simulink model "mbd_example_qdec"  (R2022b)
settings: Solver=FixedStepDiscrete  StartTime=0.0  StopTime=10.0  RelTol=1e-3  EnableMultiTasking=on
PostLoadFcn:
  | run([bdroot '_init']);
InitFcn:
  | checkModelFolder(true); % Optional
  | run([bdroot '_init']);
model workspace (MAT data in the model file):
  MBDPortal_MaskInitParam = 0
  MBDPortal_MaskInitSignal = 0
  MBDSnap_MaskInitSignal = 0
undefined symbols (not defined in the file): MBDDiag_Comm_Module, MBDDiag_Comm_Speed, MBDDiag_Comm_Type, T_s_LED1, T_s_LED2
libraries: MbdLib_PortalDiag x24, MbdLib_Uart x15, MbdLib_Digital x13, MbdLib_Qdec x10, MbdLib_Timer x8, MbdLib_SnapDiag x5, MbdLib_Sys x4, MbdLib_Required x1
settings Model: Creator=KenYoshioka  LastModifiedBy=KenYoshioka
settings SolverCC: AutoInsertRateTranBlk=on
settings OptimizationCC: DefaultParameterBehavior=Inlined  DefaultUnderspecifiedDataType=single  EnhancedBackFolding=on  BooleansAsBitfields=on  PassReuseOutputArgsAs=Individual arguments  ZeroExternalMemoryAtStartup=off  ZeroInternalMemoryAtStartup=off  OptimizeBlockOrder=speed  DifferentSizesBufferReuse=on  EfficientTunableParamExpr=on
settings DebuggingCC: MultiTaskDSMMsg=none  ParameterTunabilityLossMsg=error
settings HardwareCC: ProdBitPerPointer=32  ProdBitPerSizeT=32  ProdBitPerPtrDiffT=32  ProdLargestAtomicInteger=Long  ProdLargestAtomicFloat=Double  ProdWordSize=32  ProdHWDeviceType=ARM Compatible->ARM Cortex-M
settings ModelReferenceCC: EnableRefExpFcnMdlSchedulingChecks=on  ModelReferenceNumInstancesAllowed=Single
settings SFSimCC: MATLABDynamicMemAlloc=off
settings RTWCC: Description=MBD Embedded Target STM32 Cortex M4 (real-time)  SystemTargetFile=MBD_STM32_stf.tlc  TemplateMakefile=MBD_STM32.tmf  Toolchain=arm-none-eabi - v10.3
settings CodeAppCC: ForceParamTrailComments=on  IgnoreCustomStorageClasses=off  MaxIdLength=255  OperatorAnnotations=on  SimulinkDataObjDesc=on  SFDataObjDesc=on  InsertBlockDesc=on
settings STFCustomTargetCC: MultiwordLength=256  IncludeMdlTerminateFcn=off  CombineOutputUpdateFcns=on  CombineSignalStateStructs=on  SuppressErrorStatus=on  ERTCustomFileBanners=on  SupportContinuousTime=off  RemoveResetFunc=on  MATLABClassNameForMDSCustomization=Simulink.SoftwareTarget.ERTCustomization  UseToolchainInfoCompliant=on  SystemTargetFile=MBD_STM32_stf.tlc
settings ERTTargetCC: ParMdlRefBuildCompliant=off  CompOptLevelCompliant=off  ConcurrentExecutionCompliant=off  IncludeMdlTerminateFcn=off  CombineSignalStateStructs=on  SuppressErrorStatus=on  SupportNonInlinedSFcns=on  ModelStepFunctionPrototypeControlCompliant=off  CPPClassGenCompliant=off  ExtModeStaticAllocSize=2000  InlinedParameterPlacement=NonHierarchical  ERTCustomFileTemplate=mbd_lib_interface.tlc  MaxLineWidth=110

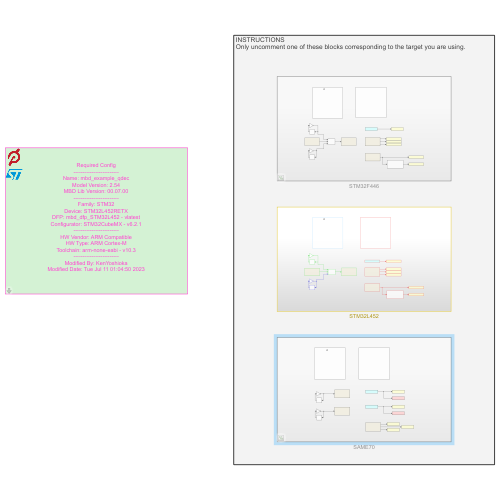
[thumbnail: Simulink's stored preview of the top-level diagram]
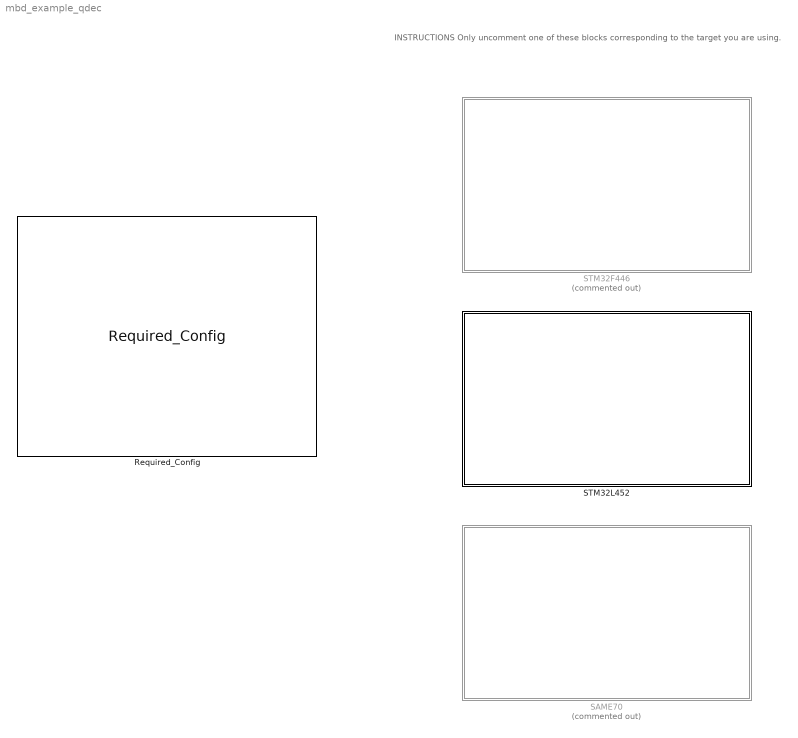
== system mbd_example_qdec ==
  note: INSTRUCTIONS
      | Only uncomment one of these blocks corresponding to the target you are using.
  Required_Config : MbdLib_Required/Required_Config  Tag=MBD_Target_Info  Param_update=1
      settings: SourceProductName=Peloton Interface Library
  SAME70 : Subsystem  Commented=on
  STM32F446 : Subsystem  Commented=on
  STM32L452 : Subsystem

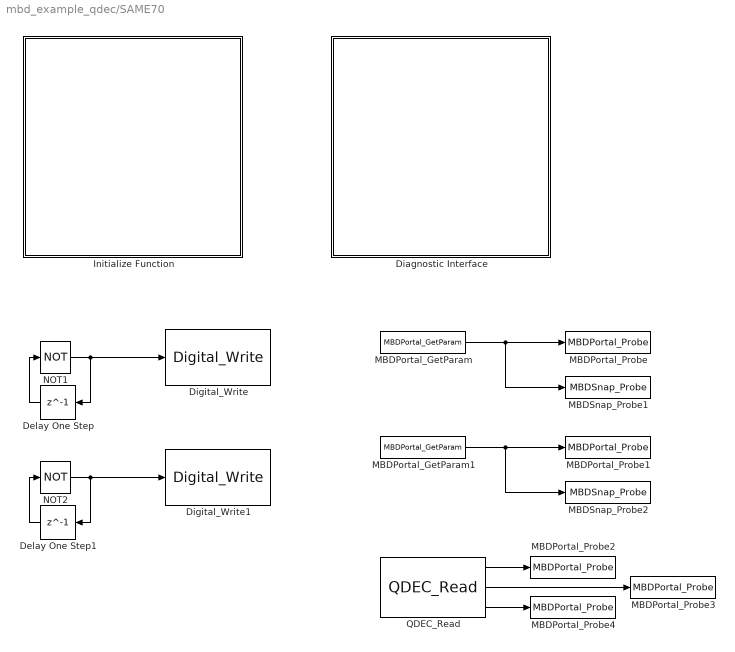
== system mbd_example_qdec/SAME70 ==
  Delay One Step : Delay  DelayLength=1  SampleTime=T_s_LED1
  Delay One Step1 : Delay  DelayLength=1  SampleTime=T_s_LED2
  Diagnostic Interface : Subsystem
  Digital_Write : MbdLib_Digital/Digital_Write  Param_module=D  Param_ch=7  Param_sampleTime=-1
      settings: SourceProductName=Peloton Interface Library
  Digital_Write1 : MbdLib_Digital/Digital_Write  Param_module=D  Param_ch=8  Param_sampleTime=-1
      settings: SourceProductName=Peloton Interface Library
  Initialize Function : Subsystem  TreatAsAtomicUnit=on
  MBDPortal_GetParam : MbdLib_PortalDiag/MBDPortal_GetParam  Param_ParamName=Parameter  Param_ParamDefault=0  Param_ParamIndex=0  Param_ParamMax=MBDPortal_ParamNum
      settings: SourceProductName=Peloton Component Library
  MBDPortal_GetParam1 : MbdLib_PortalDiag/MBDPortal_GetParam  Param_ParamName=Parameter2  Param_ParamDefault=0  Param_ParamIndex=0  Param_ParamMax=MBDPortal_ParamNum
      settings: SourceProductName=Peloton Component Library
  MBDPortal_Probe : MbdLib_PortalDiag/MBDPortal_Probe  Param_SigNameInherited=on  Param_SigName=Signals  Param_SigIndex=0  Param_SigMax=MBDPortal_SignalNum  Param_SampleTime=MBDPortal_CommonSampleRate
      settings: SourceProductName=Peloton Component Library
  MBDPortal_Probe1 : MbdLib_PortalDiag/MBDPortal_Probe  Param_SigNameInherited=on  Param_SigName=Signals2  Param_SigIndex=0  Param_SigMax=MBDPortal_SignalNum  Param_SampleTime=MBDPortal_CommonSampleRate
      settings: SourceProductName=Peloton Component Library
  MBDPortal_Probe2 : MbdLib_PortalDiag/MBDPortal_Probe  Param_SigNameInherited=on  Param_SigName=position  Param_SigIndex=0  Param_SigMax=MBDPortal_SignalNum  Param_SampleTime=MBDPortal_CommonSampleRate
      settings: SourceProductName=Peloton Component Library
  MBDPortal_Probe3 : MbdLib_PortalDiag/MBDPortal_Probe  Param_SigNameInherited=on  Param_SigName=index  Param_SigIndex=0  Param_SigMax=MBDPortal_SignalNum  Param_SampleTime=MBDPortal_CommonSampleRate
      settings: SourceProductName=Peloton Component Library
  MBDPortal_Probe4 : MbdLib_PortalDiag/MBDPortal_Probe  Param_SigNameInherited=on  Param_SigName=direction  Param_SigIndex=0  Param_SigMax=MBDPortal_SignalNum  Param_SampleTime=MBDPortal_CommonSampleRate
      settings: SourceProductName=Peloton Component Library
  MBDSnap_Probe1 : MbdLib_SnapDiag/MBDSnap_Probe  Param_SigNameInherited=on  Param_SigName=Signals  Param_SigIndex=0  Param_SigMax=MBDSnap_SignalNum  Param_StartEnable=off  Param_StartOpr=>  Param_StartThr=0  Param_StopEnable=off  Param_StopOpr=>  Param_StopThr=0  Param_StopPost=0  Param_SampleTime=MBDSnap_CommonSampleRate
      settings: SourceProductName=Peloton Component Library
  MBDSnap_Probe2 : MbdLib_SnapDiag/MBDSnap_Probe  Param_SigNameInherited=on  Param_SigName=Signals2  Param_SigIndex=0  Param_SigMax=MBDSnap_SignalNum  Param_StartEnable=off  Param_StartOpr=>  Param_StartThr=0  Param_StopEnable=off  Param_StopOpr=>  Param_StopThr=0  Param_StopPost=0  Param_SampleTime=MBDSnap_CommonSampleRate
      settings: SourceProductName=Peloton Component Library
  NOT1 : Logic  Operator=NOT  IconShape=distinctive  AllPortsSameDT=off  OutDataTypeStr=boolean
  NOT2 : Logic  Operator=NOT  IconShape=distinctive  AllPortsSameDT=off  OutDataTypeStr=boolean
  QDEC_Read : MbdLib_Qdec/QDEC_Read  Param_module=0  Param_dirOut=off  Param_sampleTime=-1  Sim_position=0  Sim_index=0  Sim_direction=0
      settings: SourceProductName=Peloton Interface Library
  wires:
  Delay One Step1/1 -> NOT2/1
  NOT1/1 -> Digital_Write/1, Delay One Step/1
  NOT2/1 -> Digital_Write1/1, Delay One Step1/1
  MBDPortal_GetParam/1 -> MBDSnap_Probe1/1, MBDPortal_Probe/1
  Delay One Step/1 -> NOT1/1
  MBDPortal_GetParam1/1 -> MBDSnap_Probe2/1, MBDPortal_Probe1/1
  QDEC_Read/2 -> MBDPortal_Probe3/1
  QDEC_Read/1 -> MBDPortal_Probe2/1
  QDEC_Read/3 -> MBDPortal_Probe4/1

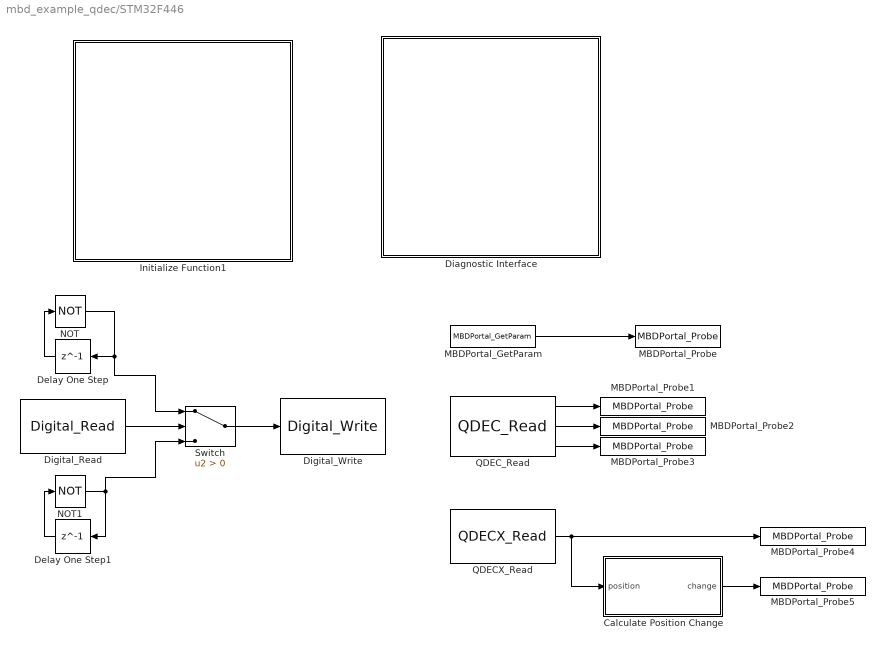
== system mbd_example_qdec/STM32F446 ==
  Calculate Position Change : Subsystem
  Delay One Step : Delay  DelayLength=1  SampleTime=T_s_LED1
  Delay One Step1 : Delay  DelayLength=1  SampleTime=T_s_LED2
  Diagnostic Interface : Subsystem
  Digital_Read : MbdLib_Digital/Digital_Read  Param_module=C  Param_ch=13  Param_sampleTime=-1  Sim_invert=off  Sim_out=0
      settings: SourceProductName=Peloton Interface Library
  Digital_Write : MbdLib_Digital/Digital_Write  Param_module=C  Param_ch=10  Param_sampleTime=-1
      settings: SourceProductName=Peloton Interface Library
  Initialize Function1 : Subsystem  TreatAsAtomicUnit=on
  MBDPortal_GetParam : MbdLib_PortalDiag/MBDPortal_GetParam  Param_ParamName=Parameter  Param_ParamDefault=0  Param_ParamIndex=0  Param_ParamMax=MBDPortal_ParamNum
      settings: SourceProductName=Peloton Component Library
  MBDPortal_Probe : MbdLib_PortalDiag/MBDPortal_Probe  Param_SigNameInherited=on  Param_SigName=Signals  Param_SigIndex=0  Param_SigMax=MBDPortal_SignalNum  Param_SampleTime=MBDPortal_CommonSampleRate
      settings: SourceProductName=Peloton Component Library
  MBDPortal_Probe1 : MbdLib_PortalDiag/MBDPortal_Probe  Param_SigNameInherited=on  Param_SigName=QDEC_position  Param_SigIndex=0  Param_SigMax=MBDPortal_SignalNum  Param_SampleTime=MBDPortal_CommonSampleRate
      settings: SourceProductName=Peloton Component Library
  MBDPortal_Probe2 : MbdLib_PortalDiag/MBDPortal_Probe  Param_SigNameInherited=on  Param_SigName=QDEC_index  Param_SigIndex=0  Param_SigMax=MBDPortal_SignalNum  Param_SampleTime=MBDPortal_CommonSampleRate
      settings: SourceProductName=Peloton Component Library
  MBDPortal_Probe3 : MbdLib_PortalDiag/MBDPortal_Probe  Param_SigNameInherited=on  Param_SigName=QDEC_direction  Param_SigIndex=0  Param_SigMax=MBDPortal_SignalNum  Param_SampleTime=MBDPortal_CommonSampleRate
      settings: SourceProductName=Peloton Component Library
  MBDPortal_Probe4 : MbdLib_PortalDiag/MBDPortal_Probe  Param_SigNameInherited=on  Param_SigName=QDECX_position  Param_SigIndex=0  Param_SigMax=MBDPortal_SignalNum  Param_SampleTime=MBDPortal_CommonSampleRate
      settings: SourceProductName=Peloton Component Library
  MBDPortal_Probe5 : MbdLib_PortalDiag/MBDPortal_Probe  Param_SigNameInherited=on  Param_SigName=QDECX_delta  Param_SigIndex=0  Param_SigMax=MBDPortal_SignalNum  Param_SampleTime=MBDPortal_CommonSampleRate
      settings: SourceProductName=Peloton Component Library
  NOT : Logic  Operator=NOT  IconShape=distinctive  AllPortsSameDT=off  OutDataTypeStr=boolean
  NOT1 : Logic  Operator=NOT  IconShape=distinctive  AllPortsSameDT=off  OutDataTypeStr=boolean
  QDECX_Read : MbdLib_Qdec/QDECX_Read  Param_module=1  Param_sampleTime=-1  Sim_position=0
      settings: SourceProductName=Peloton Interface Library
  QDEC_Read : MbdLib_Qdec/QDEC_Read  Param_module=2  Param_dirOut=off  Param_sampleTime=-1  Sim_position=0  Sim_index=0  Sim_direction=0
      settings: SourceProductName=Peloton Interface Library
  Switch : Switch  Criteria=u2 > Threshold  SaturateOnIntegerOverflow=off  InputSameDT=off
  wires:
  MBDPortal_GetParam/1 -> MBDPortal_Probe/1
  Delay One Step/1 -> NOT/1
  Digital_Read/1 -> Switch/2
  Delay One Step1/1 -> NOT1/1
  NOT1/1 -> Switch/3, Delay One Step1/1
  Switch/1 -> Digital_Write/1
  NOT/1 -> Switch/1, Delay One Step/1
  Calculate Position Change/1(change) -> MBDPortal_Probe5/1
  QDECX_Read/1 -> MBDPortal_Probe4/1, Calculate Position Change/1(position)
  QDEC_Read/2 -> MBDPortal_Probe2/1
  QDEC_Read/3 -> MBDPortal_Probe3/1
  QDEC_Read/1 -> MBDPortal_Probe1/1

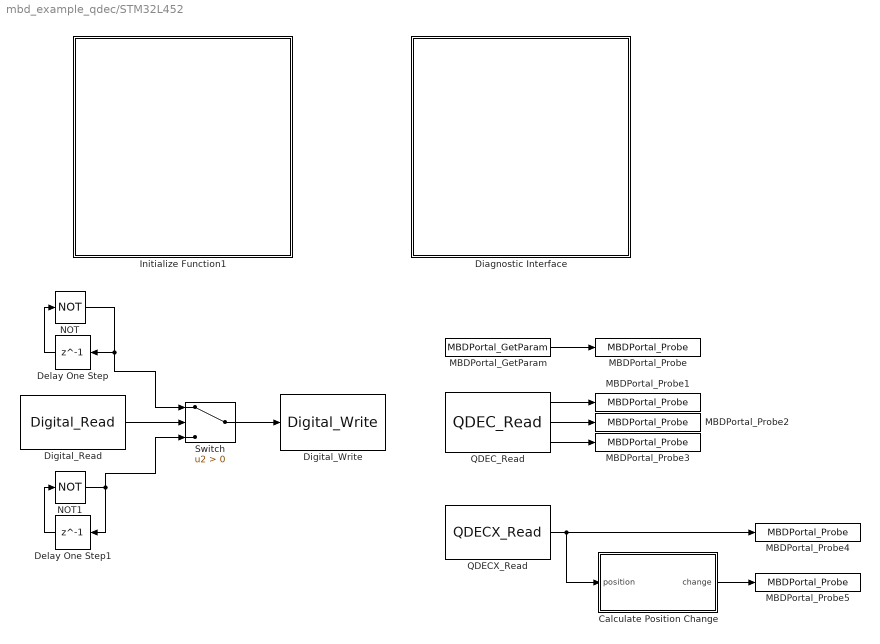
== system mbd_example_qdec/STM32L452 ==
  Calculate Position Change : Subsystem
  Delay One Step : Delay  DelayLength=1  SampleTime=T_s_LED1
  Delay One Step1 : Delay  DelayLength=1  SampleTime=T_s_LED2
  Diagnostic Interface : Subsystem
  Digital_Read : MbdLib_Digital/Digital_Read  Param_module=C  Param_ch=13  Param_sampleTime=-1  Sim_invert=off  Sim_out=0
      settings: SourceProductName=Peloton Interface Library
  Digital_Write : MbdLib_Digital/Digital_Write  Param_module=C  Param_ch=10  Param_sampleTime=-1
      settings: SourceProductName=Peloton Interface Library
  Initialize Function1 : Subsystem  TreatAsAtomicUnit=on
  MBDPortal_GetParam : MbdLib_PortalDiag/MBDPortal_GetParam  Param_ParamName=Parameter  Param_ParamDefault=0  Param_ParamIndex=0  Param_ParamMax=MBDPortal_ParamNum
      settings: SourceProductName=Peloton Component Library
  MBDPortal_Probe : MbdLib_PortalDiag/MBDPortal_Probe  Param_SigNameInherited=on  Param_SigName=Signals  Param_SigIndex=0  Param_SigMax=MBDPortal_SignalNum  Param_SampleTime=MBDPortal_CommonSampleRate
      settings: SourceProductName=Peloton Component Library
  MBDPortal_Probe1 : MbdLib_PortalDiag/MBDPortal_Probe  Param_SigNameInherited=on  Param_SigName=QDEC_position  Param_SigIndex=0  Param_SigMax=MBDPortal_SignalNum  Param_SampleTime=MBDPortal_CommonSampleRate
      settings: SourceProductName=Peloton Component Library
  MBDPortal_Probe2 : MbdLib_PortalDiag/MBDPortal_Probe  Param_SigNameInherited=on  Param_SigName=QDEC_index  Param_SigIndex=0  Param_SigMax=MBDPortal_SignalNum  Param_SampleTime=MBDPortal_CommonSampleRate
      settings: SourceProductName=Peloton Component Library
  MBDPortal_Probe3 : MbdLib_PortalDiag/MBDPortal_Probe  Param_SigNameInherited=on  Param_SigName=QDEC_direction  Param_SigIndex=0  Param_SigMax=MBDPortal_SignalNum  Param_SampleTime=MBDPortal_CommonSampleRate
      settings: SourceProductName=Peloton Component Library
  MBDPortal_Probe4 : MbdLib_PortalDiag/MBDPortal_Probe  Param_SigNameInherited=on  Param_SigName=QDECX_position  Param_SigIndex=0  Param_SigMax=MBDPortal_SignalNum  Param_SampleTime=MBDPortal_CommonSampleRate
      settings: SourceProductName=Peloton Component Library
  MBDPortal_Probe5 : MbdLib_PortalDiag/MBDPortal_Probe  Param_SigNameInherited=on  Param_SigName=QDECX_delta  Param_SigIndex=0  Param_SigMax=MBDPortal_SignalNum  Param_SampleTime=MBDPortal_CommonSampleRate
      settings: SourceProductName=Peloton Component Library
  NOT : Logic  Operator=NOT  IconShape=distinctive  AllPortsSameDT=off  OutDataTypeStr=boolean
  NOT1 : Logic  Operator=NOT  IconShape=distinctive  AllPortsSameDT=off  OutDataTypeStr=boolean
  QDECX_Read : MbdLib_Qdec/QDECX_Read  Param_module=1  Param_sampleTime=-1  Sim_position=0
      settings: SourceProductName=Peloton Interface Library
  QDEC_Read : MbdLib_Qdec/QDEC_Read  Param_module=2  Param_dirOut=off  Param_sampleTime=-1  Sim_position=0  Sim_index=0  Sim_direction=0
      settings: SourceProductName=Peloton Interface Library
  Switch : Switch  Criteria=u2 > Threshold  SaturateOnIntegerOverflow=off  InputSameDT=off
  wires:
  MBDPortal_GetParam/1 -> MBDPortal_Probe/1
  Delay One Step/1 -> NOT/1
  Digital_Read/1 -> Switch/2
  Delay One Step1/1 -> NOT1/1
  NOT1/1 -> Switch/3, Delay One Step1/1
  Switch/1 -> Digital_Write/1
  NOT/1 -> Switch/1, Delay One Step/1
  QDEC_Read/1 -> MBDPortal_Probe1/1
  QDEC_Read/2 -> MBDPortal_Probe2/1
  QDEC_Read/3 -> MBDPortal_Probe3/1
  QDECX_Read/1 -> MBDPortal_Probe4/1, Calculate Position Change/1(position)
  Calculate Position Change/1(change) -> MBDPortal_Probe5/1

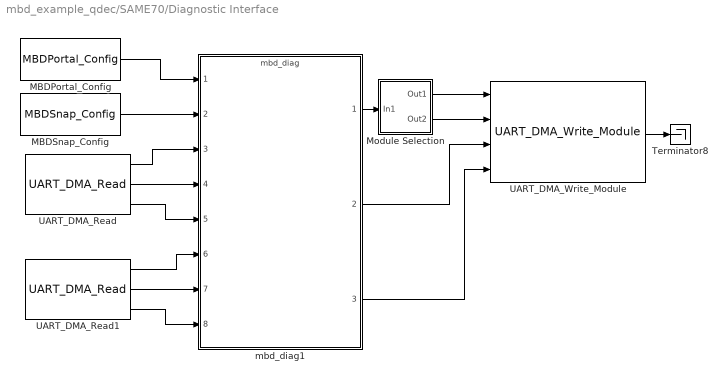
== system mbd_example_qdec/SAME70/Diagnostic Interface ==
  MBDPortal_Config : MbdLib_PortalDiag/MBDPortal_Config  Param_SigMax=MBDPortal_SignalNum  Param_ParamMax=MBDPortal_ParamNum
      settings: SourceProductName=Peloton Component Library
  MBDSnap_Config : MbdLib_SnapDiag/MBDSnap_Config  Priority=-5000  Param_enableAll=on  Param_SampleTime=T_s_COMM  Param_SigMax=MBDSnap_SignalNum
      settings: SourceProductName=Peloton Component Library
  Module Selection : Subsystem
  Terminator8 : Terminator
  UART_DMA_Read : MbdLib_Uart/UART_DMA_Read  Tag=TAG_UART_DMA  Param_module=MBDDiag_Comm_Module(1)  Param_type=USART  Param_readLim=100  Param_sampleTime=T_s_COMM
      settings: SourceProductName=Peloton Interface Library
  UART_DMA_Read1 : MbdLib_Uart/UART_DMA_Read  Tag=TAG_UART_DMA  Param_module=MBDDiag_Comm_Module(2)  Param_type=USART  Param_readLim=100  Param_sampleTime=T_s_COMM
      settings: SourceProductName=Peloton Interface Library
  UART_DMA_Write_Module : MbdLib_Uart/UART_DMA_Write_Module  Param_instanceNum=2  Param_module1=MBDDiag_Comm_Module(1)  Param_type1=USART  Param_module2=MBDDiag_Comm_Module(2)  Param_type2=USART  Param_module3=0  Param_type3=UART  Param_module4=0  Param_type4=UART  Param_sampleTime=-1  Sim_status=0
      settings: SourceProductName=Peloton Interface Library
  mbd_diag1 : ModelReference  ModelNameDialog=mbd_diag.slx  SimulationMode=Normal  ModelReferenceVersion=2.292  SimulationMode=Normal
  wires:
  Module Selection/2(Out2) -> UART_DMA_Write_Module/2
  UART_DMA_Read1/2 -> mbd_diag1/7
  UART_DMA_Read/1 -> mbd_diag1/3
  UART_DMA_Write_Module/1 -> Terminator8/1
  mbd_diag1/1 -> Module Selection/1(In1)
  MBDPortal_Config/1 -> mbd_diag1/1
  mbd_diag1/3 -> UART_DMA_Write_Module/4
  MBDSnap_Config/1 -> mbd_diag1/2
  mbd_diag1/2 -> UART_DMA_Write_Module/3
  UART_DMA_Read/2 -> mbd_diag1/4
  Module Selection/1(Out1) -> UART_DMA_Write_Module/1
  UART_DMA_Read1/1 -> mbd_diag1/6
  UART_DMA_Read/3 -> mbd_diag1/5
  UART_DMA_Read1/3 -> mbd_diag1/8

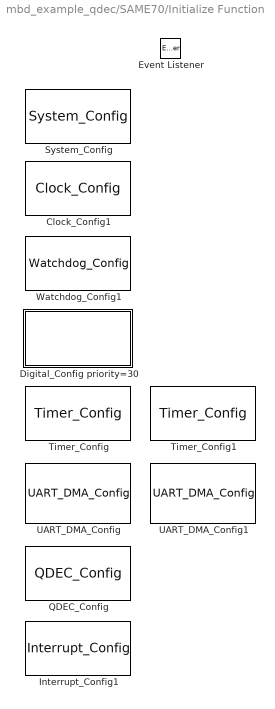
== system mbd_example_qdec/SAME70/Initialize Function ==
  Clock_Config1 : MbdLib_Sys/Clock_Config  Priority=10  Param_frequency=Peripheral_Clock_Hz  Param_priority=10  Param_sampleTime=-1
      settings: AttributesFormatString=priority=%<priority>  SourceProductName=Peloton Interface Library
  Digital_Config priority=30 : Subsystem
  Event Listener : EventListener  DisableCoverage=on  EventName=reset
  Interrupt_Config1 : MbdLib_Sys/Interrupt_Config  Priority=120  Param_priority=120  Param_sampleTime=-1
      settings: AttributesFormatString=priority=%<priority>  SourceProductName=Peloton Interface Library
  QDEC_Config : MbdLib_Qdec/QDEC_Config  Priority=110  Param_module=0  Param_priority=110  Param_sampleTime=-1
      settings: AttributesFormatString=priority=%<priority>  SourceProductName=Peloton Interface Library
  System_Config : MbdLib_Sys/System_Config  Priority=0  Param_priority=0  Param_sampleTime=-1
      settings: AttributesFormatString=priority=%<priority>  SourceProductName=Peloton Interface Library
  Timer_Config : MbdLib_Timer/Timer_Config  Priority=100  Param_update=1  Param_module=2  Param_step=0  Param_period=Base_period_cycles  Param_divider=0  Param_step0=0  Param_clksrc0=1  Param_period0=Base_period_cycles  Param_divider0=0  Param_step1=1  Param_clksrc1=1  Param_period1=Comm_period_cycles  Param_divider1=0  Param_step2=2  Param_clksrc2=2  Param_period2=LED1_period_cycles  Param_divider2=0  Param_priority=100  Param_sampleTime=-1
      settings: AttributesFormatString=priority=%<priority>  SourceProductName=Peloton Interface Library
  Timer_Config1 : MbdLib_Timer/Timer_Config  Priority=100  Param_update=1  Param_module=3  Param_step=3  Param_period=LED2_period_cycles  Param_divider=0  Param_step0=3  Param_clksrc0=2  Param_period0=LED2_period_cycles  Param_divider0=0  Param_step1=-1  Param_clksrc1=0  Param_period1=0  Param_divider1=0  Param_step2=-1  Param_clksrc2=0  Param_period2=0  Param_divider2=0  Param_priority=100  Param_sampleTime=-1
      settings: AttributesFormatString=priority=%<priority>  SourceProductName=Peloton Interface Library
  UART_DMA_Config : MbdLib_Uart/UART_DMA_Config  Priority=110  Param_module=MBDDiag_Comm_Module(1)  Param_type=USART  Param_speed=MBDDiag_Comm_Speed(1)  Param_dataBits=8  Param_stopBits=0.5  Param_parity=None  Param_priority=110  Param_sampleTime=-1
      settings: AttributesFormatString=priority=%<priority>  SourceProductName=Peloton Interface Library
  UART_DMA_Config1 : MbdLib_Uart/UART_DMA_Config  Priority=110  Param_module=MBDDiag_Comm_Module(2)  Param_type=USART  Param_speed=MBDDiag_Comm_Speed(2)  Param_dataBits=8  Param_stopBits=0.5  Param_parity=None  Param_priority=110  Param_sampleTime=-1
      settings: AttributesFormatString=priority=%<priority>  SourceProductName=Peloton Interface Library
  Watchdog_Config1 : MbdLib_Sys/Watchdog_Config  Priority=20  Param_enable=off  Param_priority=20  Param_sampleTime=-1
      settings: AttributesFormatString=priority=%<priority>  SourceProductName=Peloton Interface Library

== system mbd_example_qdec/STM32F446/Calculate Position Change ==
  position : Inport
  Data Type Conversion : DataTypeConversion  OutDataTypeStr=int32  ConvertRealWorld=Stored Integer (SI)  SaturateOnIntegerOverflow=off  RndMeth=Floor
  Delay One Step2 : Delay  DelayLength=1
  Subtract : Sum  Inputs=+-
  change : Outport
  wires:
  Delay One Step2/1 -> Subtract/2
  position/1 -> Delay One Step2/1, Subtract/1
  Subtract/1 -> Data Type Conversion/1
  Data Type Conversion/1 -> change/1

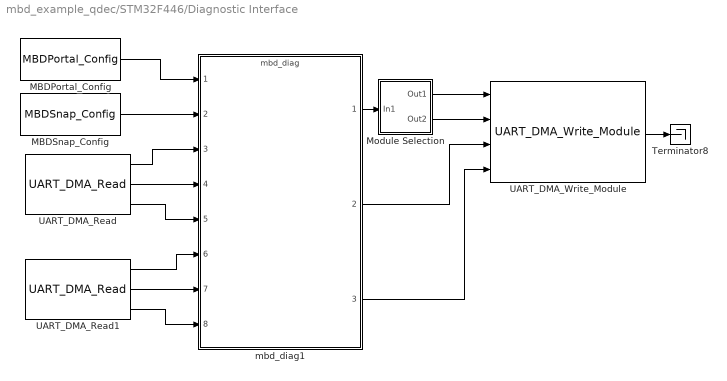
== system mbd_example_qdec/STM32F446/Diagnostic Interface ==
  MBDPortal_Config : MbdLib_PortalDiag/MBDPortal_Config  Param_SigMax=MBDPortal_SignalNum  Param_ParamMax=MBDPortal_ParamNum
      settings: SourceProductName=Peloton Component Library
  MBDSnap_Config : MbdLib_SnapDiag/MBDSnap_Config  Priority=-5000  Param_enableAll=on  Param_SampleTime=T_s_COMM  Param_SigMax=MBDSnap_SignalNum
      settings: SourceProductName=Peloton Component Library
  Module Selection : Subsystem
  Terminator8 : Terminator
  UART_DMA_Read : MbdLib_Uart/UART_DMA_Read  Tag=TAG_UART_DMA  Param_module=MBDDiag_Comm_Module(1)  Param_type=USART  Param_readLim=100  Param_sampleTime=T_s_COMM
      settings: SourceProductName=Peloton Interface Library
  UART_DMA_Read1 : MbdLib_Uart/UART_DMA_Read  Tag=TAG_UART_DMA  Param_module=MBDDiag_Comm_Module(2)  Param_type=USART  Param_readLim=100  Param_sampleTime=T_s_COMM
      settings: SourceProductName=Peloton Interface Library
  UART_DMA_Write_Module : MbdLib_Uart/UART_DMA_Write_Module  Param_instanceNum=2  Param_module1=MBDDiag_Comm_Module(1)  Param_type1=USART  Param_module2=MBDDiag_Comm_Module(2)  Param_type2=USART  Param_module3=0  Param_type3=UART  Param_module4=0  Param_type4=UART  Param_sampleTime=-1  Sim_status=0
      settings: SourceProductName=Peloton Interface Library
  mbd_diag1 : ModelReference  ModelNameDialog=mbd_diag.slx  SimulationMode=Normal  ModelReferenceVersion=2.292  SimulationMode=Normal
  wires:
  Module Selection/2(Out2) -> UART_DMA_Write_Module/2
  UART_DMA_Read1/2 -> mbd_diag1/7
  UART_DMA_Read/1 -> mbd_diag1/3
  UART_DMA_Write_Module/1 -> Terminator8/1
  mbd_diag1/1 -> Module Selection/1(In1)
  MBDPortal_Config/1 -> mbd_diag1/1
  mbd_diag1/3 -> UART_DMA_Write_Module/4
  MBDSnap_Config/1 -> mbd_diag1/2
  mbd_diag1/2 -> UART_DMA_Write_Module/3
  UART_DMA_Read/2 -> mbd_diag1/4
  Module Selection/1(Out1) -> UART_DMA_Write_Module/1
  UART_DMA_Read1/1 -> mbd_diag1/6
  UART_DMA_Read/3 -> mbd_diag1/5
  UART_DMA_Read1/3 -> mbd_diag1/8

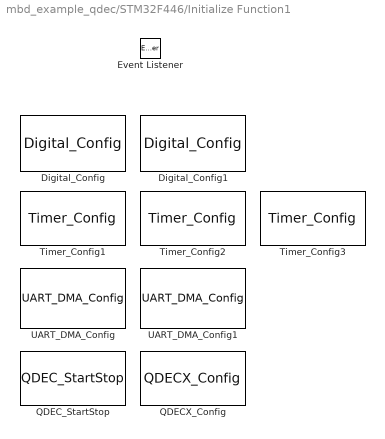
== system mbd_example_qdec/STM32F446/Initialize Function1 ==
  Digital_Config : MbdLib_Digital/Digital_Config  Priority=30  Param_module=C  Param_ch=10  Param_dir=output  Param_pupd=none  Param_default=low  Param_mode=none  Param_drive=low  Param_speed=high  Param_priority=30  Param_sampleTime=-1
      settings: AttributesFormatString=priority=%<priority>  SourceProductName=Peloton Interface Library
  Digital_Config1 : MbdLib_Digital/Digital_Config  Priority=30  Param_module=C  Param_ch=13  Param_dir=input  Param_pupd=pullup  Param_default=low  Param_mode=none  Param_drive=low  Param_speed=high  Param_priority=30  Param_sampleTime=-1
      settings: AttributesFormatString=priority=%<priority>  SourceProductName=Peloton Interface Library
  Event Listener : EventListener  DisableCoverage=on  EventName=reset
  QDECX_Config : MbdLib_Qdec/QDECX_Config  Priority=120  Param_module=1  Param_portA=B  Param_pinA=10  Param_portB=B  Param_pinB=11  Param_priority=120  Param_sampleTime=-1
      settings: AttributesFormatString=priority=%<priority>  SourceProductName=Peloton Interface Library
  QDEC_StartStop : MbdLib_Qdec/QDEC_StartStop  Priority=120  Param_module=2  Param_action=Start  Param_priority=120  Param_sampleTime=-1
      settings: AttributesFormatString=priority=%<priority>  SourceProductName=Peloton Interface Library
  Timer_Config1 : MbdLib_Timer/Timer_Config  Priority=100  Param_update=1  Param_module=1  Param_step=0  Param_period=Comm_period_cycles  Param_divider=Comm_clock_divider  Param_step0=0  Param_clksrc0=0  Param_period0=Comm_period_cycles  Param_divider0=Comm_clock_divider  Param_step1=-1  Param_clksrc1=0  Param_period1=0  Param_divider1=0  Param_step2=-1  Param_clksrc2=0  Param_period2=0  Param_divider2=0  Param_priority=100  Param_sampleTime=-1
      settings: AttributesFormatString=priority=%<priority>  SourceProductName=Peloton Interface Library
  Timer_Config2 : MbdLib_Timer/Timer_Config  Priority=101  Param_update=1  Param_module=6  Param_step=1  Param_period=LED1_period_cycles  Param_divider=LED1_clock_divider  Param_step0=1  Param_clksrc0=0  Param_period0=LED1_period_cycles  Param_divider0=LED1_clock_divider  Param_step1=-1  Param_clksrc1=0  Param_period1=0  Param_divider1=0  Param_step2=-1  Param_clksrc2=0  Param_period2=0  Param_divider2=0  Param_priority=101  Param_sampleTime=-1
      settings: AttributesFormatString=priority=%<priority>  SourceProductName=Peloton Interface Library
  Timer_Config3 : MbdLib_Timer/Timer_Config  Priority=102  Param_update=1  Param_module=7  Param_step=2  Param_period=LED2_period_cycles  Param_divider=LED2_clock_divider  Param_step0=2  Param_clksrc0=0  Param_period0=LED2_period_cycles  Param_divider0=LED2_clock_divider  Param_step1=-1  Param_clksrc1=0  Param_period1=0  Param_divider1=0  Param_step2=-1  Param_clksrc2=0  Param_period2=0  Param_divider2=0  Param_priority=102  Param_sampleTime=-1
      settings: AttributesFormatString=priority=%<priority>  SourceProductName=Peloton Interface Library
  UART_DMA_Config : MbdLib_Uart/UART_DMA_Config  Priority=110  Param_module=MBDDiag_Comm_Module(1)  Param_type=USART  Param_speed=MBDDiag_Comm_Speed(1)  Param_dataBits=8  Param_stopBits=1  Param_parity=None  Param_priority=110  Param_sampleTime=-1
      settings: AttributesFormatString=priority=%<priority>  SourceProductName=Peloton Interface Library
  UART_DMA_Config1 : MbdLib_Uart/UART_DMA_Config  Priority=110  Param_module=MBDDiag_Comm_Module(2)  Param_type=USART  Param_speed=MBDDiag_Comm_Speed(2)  Param_dataBits=8  Param_stopBits=1  Param_parity=None  Param_priority=110  Param_sampleTime=-1
      settings: AttributesFormatString=priority=%<priority>  SourceProductName=Peloton Interface Library

== system mbd_example_qdec/STM32L452/Calculate Position Change ==
  position : Inport
  Data Type Conversion : DataTypeConversion  OutDataTypeStr=int32  ConvertRealWorld=Stored Integer (SI)  SaturateOnIntegerOverflow=off  RndMeth=Floor
  Delay One Step2 : Delay  DelayLength=1
  Subtract : Sum  Inputs=+-
  change : Outport
  wires:
  Delay One Step2/1 -> Subtract/2
  position/1 -> Delay One Step2/1, Subtract/1
  Subtract/1 -> Data Type Conversion/1
  Data Type Conversion/1 -> change/1

== system mbd_example_qdec/STM32L452/Diagnostic Interface ==
  MBDPortal_Config : MbdLib_PortalDiag/MBDPortal_Config  Param_SigMax=MBDPortal_SignalNum  Param_ParamMax=MBDPortal_ParamNum
      settings: SourceProductName=Peloton Component Library
  MBDSnap_Config : MbdLib_SnapDiag/MBDSnap_Config  Priority=-5000  Param_enableAll=on  Param_SampleTime=T_s_COMM  Param_SigMax=MBDSnap_SignalNum
      settings: SourceProductName=Peloton Component Library
  Module Selection : Subsystem
  Terminator8 : Terminator
  UART_DMA_Read : MbdLib_Uart/UART_DMA_Read  Tag=TAG_UART_DMA  Param_module=MBDDiag_Comm_Module(1)  Param_type=USART  Param_readLim=100  Param_sampleTime=T_s_COMM
      settings: SourceProductName=Peloton Interface Library
  UART_DMA_Read1 : MbdLib_Uart/UART_DMA_Read  Tag=TAG_UART_DMA  Param_module=MBDDiag_Comm_Module(2)  Param_type=USART  Param_readLim=100  Param_sampleTime=T_s_COMM
      settings: SourceProductName=Peloton Interface Library
  UART_DMA_Write_Module : MbdLib_Uart/UART_DMA_Write_Module  Param_instanceNum=2  Param_module1=MBDDiag_Comm_Module(1)  Param_type1=USART  Param_module2=MBDDiag_Comm_Module(2)  Param_type2=USART  Param_module3=0  Param_type3=UART  Param_module4=0  Param_type4=UART  Param_sampleTime=-1  Sim_status=0
      settings: SourceProductName=Peloton Interface Library
  mbd_diag1 : ModelReference  ModelNameDialog=mbd_diag.slx  SimulationMode=Normal  ModelReferenceVersion=2.292  SimulationMode=Normal
  wires:
  Module Selection/2(Out2) -> UART_DMA_Write_Module/2
  UART_DMA_Read1/2 -> mbd_diag1/7
  UART_DMA_Read/1 -> mbd_diag1/3
  UART_DMA_Write_Module/1 -> Terminator8/1
  mbd_diag1/1 -> Module Selection/1(In1)
  MBDPortal_Config/1 -> mbd_diag1/1
  mbd_diag1/3 -> UART_DMA_Write_Module/4
  MBDSnap_Config/1 -> mbd_diag1/2
  mbd_diag1/2 -> UART_DMA_Write_Module/3
  UART_DMA_Read/2 -> mbd_diag1/4
  Module Selection/1(Out1) -> UART_DMA_Write_Module/1
  UART_DMA_Read1/1 -> mbd_diag1/6
  UART_DMA_Read/3 -> mbd_diag1/5
  UART_DMA_Read1/3 -> mbd_diag1/8

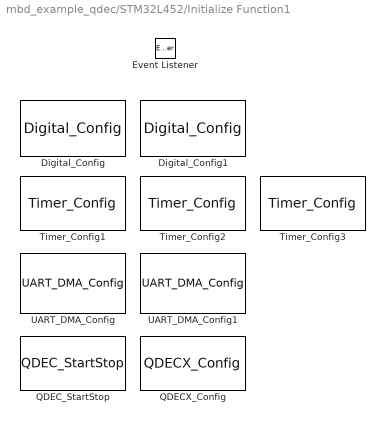
== system mbd_example_qdec/STM32L452/Initialize Function1 ==
  Digital_Config : MbdLib_Digital/Digital_Config  Priority=30  Param_module=C  Param_ch=10  Param_dir=output  Param_pupd=none  Param_default=low  Param_mode=none  Param_drive=low  Param_speed=high  Param_priority=30  Param_sampleTime=-1
      settings: AttributesFormatString=priority=%<priority>  SourceProductName=Peloton Interface Library
  Digital_Config1 : MbdLib_Digital/Digital_Config  Priority=30  Param_module=C  Param_ch=13  Param_dir=input  Param_pupd=pullup  Param_default=low  Param_mode=none  Param_drive=low  Param_speed=high  Param_priority=30  Param_sampleTime=-1
      settings: AttributesFormatString=priority=%<priority>  SourceProductName=Peloton Interface Library
  Event Listener : EventListener  DisableCoverage=on  EventName=reset
  QDECX_Config : MbdLib_Qdec/QDECX_Config  Priority=120  Param_module=1  Param_portA=B  Param_pinA=10  Param_portB=B  Param_pinB=11  Param_priority=120  Param_sampleTime=-1
      settings: AttributesFormatString=priority=%<priority>  SourceProductName=Peloton Interface Library
  QDEC_StartStop : MbdLib_Qdec/QDEC_StartStop  Priority=120  Param_module=2  Param_action=Start  Param_priority=120  Param_sampleTime=-1
      settings: AttributesFormatString=priority=%<priority>  SourceProductName=Peloton Interface Library
  Timer_Config1 : MbdLib_Timer/Timer_Config  Priority=100  Param_update=1  Param_module=6  Param_step=0  Param_period=Comm_period_cycles  Param_divider=Comm_clock_divider  Param_step0=0  Param_clksrc0=0  Param_period0=Comm_period_cycles  Param_divider0=Comm_clock_divider  Param_step1=-1  Param_clksrc1=0  Param_period1=0  Param_divider1=0  Param_step2=-1  Param_clksrc2=0  Param_period2=0  Param_divider2=0  Param_priority=100  Param_sampleTime=-1
      settings: AttributesFormatString=priority=%<priority>  SourceProductName=Peloton Interface Library
  Timer_Config2 : MbdLib_Timer/Timer_Config  Priority=101  Param_update=1  Param_module=15  Param_step=1  Param_period=LED1_period_cycles  Param_divider=LED1_clock_divider  Param_step0=1  Param_clksrc0=0  Param_period0=LED1_period_cycles  Param_divider0=LED1_clock_divider  Param_step1=-1  Param_clksrc1=0  Param_period1=0  Param_divider1=0  Param_step2=-1  Param_clksrc2=0  Param_period2=0  Param_divider2=0  Param_priority=101  Param_sampleTime=-1
      settings: AttributesFormatString=priority=%<priority>  SourceProductName=Peloton Interface Library
  Timer_Config3 : MbdLib_Timer/Timer_Config  Priority=102  Param_update=1  Param_module=16  Param_step=2  Param_period=LED2_period_cycles  Param_divider=LED2_clock_divider  Param_step0=2  Param_clksrc0=0  Param_period0=LED2_period_cycles  Param_divider0=LED2_clock_divider  Param_step1=-1  Param_clksrc1=0  Param_period1=0  Param_divider1=0  Param_step2=-1  Param_clksrc2=0  Param_period2=0  Param_divider2=0  Param_priority=102  Param_sampleTime=-1
      settings: AttributesFormatString=priority=%<priority>  SourceProductName=Peloton Interface Library
  UART_DMA_Config : MbdLib_Uart/UART_DMA_Config  Priority=110  Param_module=MBDDiag_Comm_Module(1)  Param_type=USART  Param_speed=MBDDiag_Comm_Speed(1)  Param_dataBits=8  Param_stopBits=1  Param_parity=None  Param_priority=110  Param_sampleTime=-1
      settings: AttributesFormatString=priority=%<priority>  SourceProductName=Peloton Interface Library
  UART_DMA_Config1 : MbdLib_Uart/UART_DMA_Config  Priority=110  Param_module=MBDDiag_Comm_Module(2)  Param_type=USART  Param_speed=MBDDiag_Comm_Speed(2)  Param_dataBits=8  Param_stopBits=1  Param_parity=None  Param_priority=110  Param_sampleTime=-1
      settings: AttributesFormatString=priority=%<priority>  SourceProductName=Peloton Interface Library

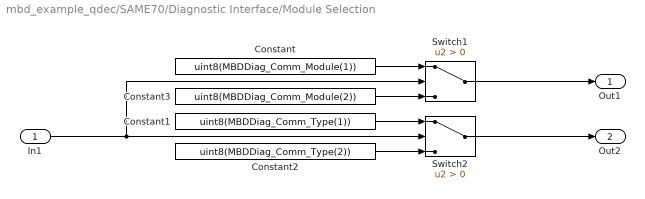
== system mbd_example_qdec/SAME70/Diagnostic Interface/Module Selection ==
  In1 : Inport
  Constant : Constant  Value=uint8(MBDDiag_Comm_Module(1))
  Constant1 : Constant  Value=uint8(MBDDiag_Comm_Type(1))
  Constant2 : Constant  Value=uint8(MBDDiag_Comm_Type(2))
  Constant3 : Constant  Value=uint8(MBDDiag_Comm_Module(2))
  Switch1 : Switch  Criteria=u2 > Threshold  SaturateOnIntegerOverflow=off  InputSameDT=off
  Switch2 : Switch  Criteria=u2 > Threshold  SaturateOnIntegerOverflow=off  InputSameDT=off
  Out1 : Outport
  Out2 : Outport  Port=2
  wires:
  In1/1 -> Switch1/2, Switch2/2
  Constant3/1 -> Switch1/3
  Switch1/1 -> Out1/1
  Constant/1 -> Switch1/1
  Constant1/1 -> Switch2/1
  Switch2/1 -> Out2/1
  Constant2/1 -> Switch2/3

== system mbd_example_qdec/SAME70/Initialize Function/Digital_Config priority=30 ==
  Digital_Config : MbdLib_Digital/Digital_Config  Priority=0  Param_module=D  Param_ch=7  Param_dir=output  Param_pupd=none  Param_default=low  Param_mode=none  Param_drive=low  Param_speed=low  Param_priority=0  Param_sampleTime=-1
      settings: SourceProductName=Peloton Interface Library
  Digital_Config1 : MbdLib_Digital/Digital_Config  Priority=0  Param_module=D  Param_ch=8  Param_dir=output  Param_pupd=none  Param_default=low  Param_mode=none  Param_drive=low  Param_speed=low  Param_priority=0  Param_sampleTime=-1
      settings: SourceProductName=Peloton Interface Library
  Digital_Config2 : MbdLib_Digital/Digital_Config  Priority=0  Param_module=D  Param_ch=9  Param_dir=output  Param_pupd=none  Param_default=low  Param_mode=none  Param_drive=low  Param_speed=low  Param_priority=0  Param_sampleTime=-1
      settings: SourceProductName=Peloton Interface Library

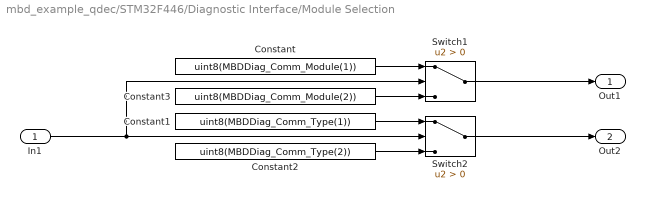
== system mbd_example_qdec/STM32F446/Diagnostic Interface/Module Selection ==
  In1 : Inport
  Constant : Constant  Value=uint8(MBDDiag_Comm_Module(1))
  Constant1 : Constant  Value=uint8(MBDDiag_Comm_Type(1))
  Constant2 : Constant  Value=uint8(MBDDiag_Comm_Type(2))
  Constant3 : Constant  Value=uint8(MBDDiag_Comm_Module(2))
  Switch1 : Switch  Criteria=u2 > Threshold  SaturateOnIntegerOverflow=off  InputSameDT=off
  Switch2 : Switch  Criteria=u2 > Threshold  SaturateOnIntegerOverflow=off  InputSameDT=off
  Out1 : Outport
  Out2 : Outport  Port=2
  wires:
  In1/1 -> Switch1/2, Switch2/2
  Constant3/1 -> Switch1/3
  Switch1/1 -> Out1/1
  Constant/1 -> Switch1/1
  Constant1/1 -> Switch2/1
  Switch2/1 -> Out2/1
  Constant2/1 -> Switch2/3

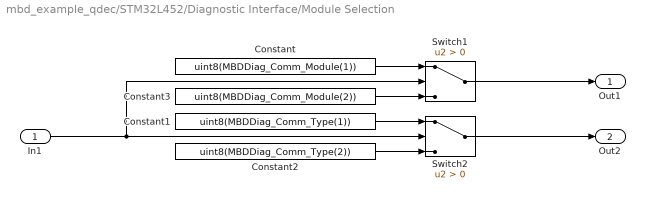
== system mbd_example_qdec/STM32L452/Diagnostic Interface/Module Selection ==
  In1 : Inport
  Constant : Constant  Value=uint8(MBDDiag_Comm_Module(1))
  Constant1 : Constant  Value=uint8(MBDDiag_Comm_Type(1))
  Constant2 : Constant  Value=uint8(MBDDiag_Comm_Type(2))
  Constant3 : Constant  Value=uint8(MBDDiag_Comm_Module(2))
  Switch1 : Switch  Criteria=u2 > Threshold  SaturateOnIntegerOverflow=off  InputSameDT=off
  Switch2 : Switch  Criteria=u2 > Threshold  SaturateOnIntegerOverflow=off  InputSameDT=off
  Out1 : Outport
  Out2 : Outport  Port=2
  wires:
  In1/1 -> Switch1/2, Switch2/2
  Constant3/1 -> Switch1/3
  Switch1/1 -> Out1/1
  Constant/1 -> Switch1/1
  Constant1/1 -> Switch2/1
  Switch2/1 -> Out2/1
  Constant2/1 -> Switch2/3
